simulink library "bonsai_library"  (R2020b)
settings: Solver=VariableStepAuto  StartTime=0.0  StopTime=10.0  RelTol=1e-3
settings Model: Creator=skamacpro  LastModifiedBy=navvaranmann

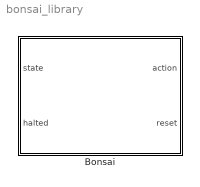
== system bonsai_library ==
  Bonsai : MATLAB Function  TreatAsAtomicUnit=on

== matlab function bonsai_library/Bonsai ==
  data: state input; action output; halted input; reset output
function [action, reset]= fcn(state, halted)
end
